simulink model "SquareWaveSumOfSineWaves"  (R2015b)
settings: Solver=VariableStepAuto  StartTime=0.0  StopTime=10.0  MaxStep=0.001  MinStep=0.001  RelTol=1e-3
settings Model: Creator=mihai.ciobanu  LastModifiedBy=mihai.ciobanu

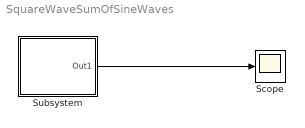
== system SquareWaveSumOfSineWaves ==
  Scope : Scope
  Subsystem : Subsystem
  wires:
  Subsystem/1(Out1) -> Scope/1

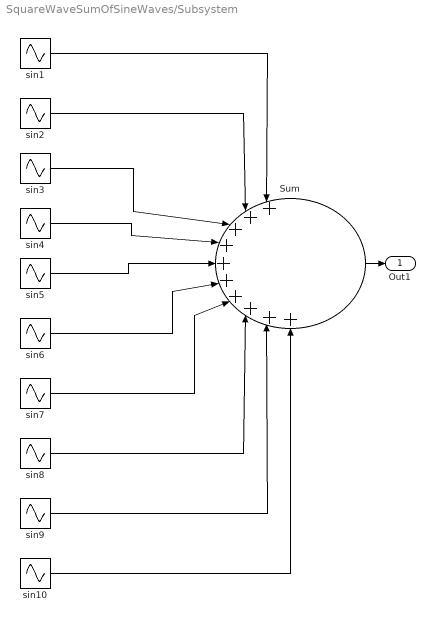
== system SquareWaveSumOfSineWaves/Subsystem ==
  Sum : Sum  Inputs=|++++++++++
  sin1 : Sin  SampleTime=0
  sin10 : Sin  Amplitude=1/19  Frequency=19  SampleTime=0
  sin2 : Sin  Amplitude=1/3  Frequency=3  SampleTime=0
  sin3 : Sin  Amplitude=1/5  Frequency=5  SampleTime=0
  sin4 : Sin  Amplitude=1/7  Frequency=7  SampleTime=0
  sin5 : Sin  Amplitude=1/9  Frequency=9  SampleTime=0
  sin6 : Sin  Amplitude=1/11  Frequency=11  SampleTime=0
  sin7 : Sin  Amplitude=1/13  Frequency=13  SampleTime=0
  sin8 : Sin  Amplitude=1/15  Frequency=15  SampleTime=0
  sin9 : Sin  Amplitude=1/17  Frequency=17  SampleTime=0
  Out1 : Outport
  wires:
  Sum/1 -> Out1/1
  sin1/1 -> Sum/1
  sin2/1 -> Sum/2
  sin5/1 -> Sum/5
  sin4/1 -> Sum/4
  sin9/1 -> Sum/9
  sin3/1 -> Sum/3
  sin8/1 -> Sum/8
  sin10/1 -> Sum/10
  sin7/1 -> Sum/7
  sin6/1 -> Sum/6
